simulink model "model"  (R2022a)
settings: Solver=VariableStepAuto  StartTime=0.0  StopTime=Inf  RelTol=1e-3
settings Model: Creator=mateu  LastModifiedBy=mateu

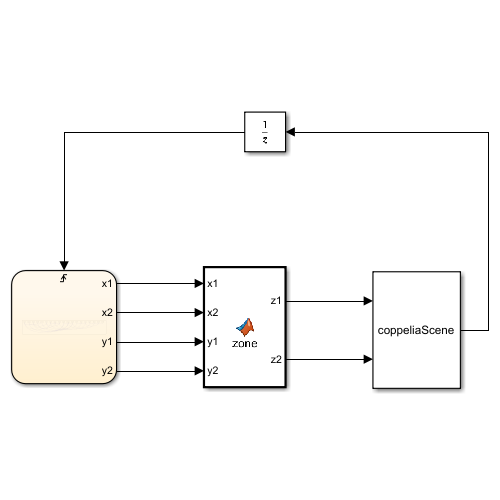
[thumbnail: Simulink's stored preview of the top-level diagram]
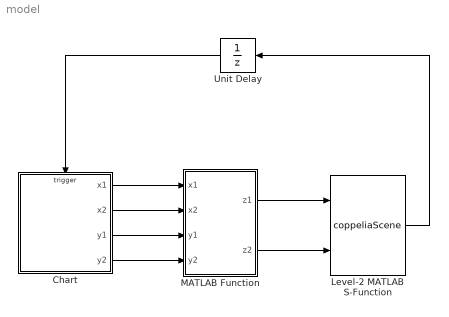
== system model ==
  Chart : Stateflow chart  TreatAsAtomicUnit=on
  Level-2 MATLAB S-Function : M-S-Function  FunctionName=coppeliaScene
  MATLAB Function : MATLAB Function  TreatAsAtomicUnit=on
  Unit Delay : UnitDelay  SampleTime=-1  HasFrameUpgradeWarning=on
  wires:
  MATLAB Function/2(z2) -> Level-2 MATLAB S-Function/2
  MATLAB Function/1(z1) -> Level-2 MATLAB S-Function/1
  Level-2 MATLAB S-Function/1 -> Unit Delay/1
  Chart/1(x1) -> MATLAB Function/1(x1)
  Chart/3(y1) -> MATLAB Function/3(y1)
  Chart/2(x2) -> MATLAB Function/2(x2)
  Chart/4(y2) -> MATLAB Function/4(y2)
  Unit Delay/1 -> Chart/Trigger

== matlab function model/MATLAB Function ==
  data: x1 input; x2 input; z1 output; y1 input; y2 input; z2 output
function [z1,z2] = zone(x1,x2,y1,y2)

z1 = x1 + (y1-1)*3;
z2 = x2 + (y2-1)*3;

== stateflow chart model/Chart ==
  settings: executeAtInitialization=1
  state R_1__x__R_1__y__R_2__x__R_2__y__sup_R_1__S_D__R_1__S_L__R_1__S_R__R_1__S_U__R_1__x__R_1__y__R_2__S_D__R_2__S_L__R_2__S_R__R_2__S_U__R_2__x__R_2__y__S_Collision__S_Task_1___S_Task_2__
    state s01
      x1=1;
      y1=1;
      x2=1;
      y2=2;
    state s02
      x1=1;
      y1=1;
      x2=1;
      y2=2;
    state s03
      x1=1;
      y1=1;
      x2=1;
      y2=3;
    state s04
      x1=1;
      y1=1;
      x2=1;
      y2=3;
    state s05
      x1=1;
      y1=1;
      x2=2;
      y2=1;
    state s06
      x1=1;
      y1=1;
      x2=2;
      y2=1;
    state s07
      x1=1;
      y1=1;
      x2=2;
      y2=1;
    state s08
      x1=1;
      y1=1;
      x2=2;
      y2=2;
    state s09
      x1=1;
      y1=1;
      x2=2;
      y2=2;
    state s010
      x1=1;
      y1=1;
      x2=2;
      y2=3;
    state s011
      x1=1;
      y1=1;
      x2=2;
      y2=3;
    state s012
      x1=1;
      y1=1;
      x2=2;
      y2=3;
    state s013
      x1=1;
      y1=1;
      x2=2;
      y2=3;
    state s014
      x1=1;
      y1=1;
      x2=3;
      y2=1;
    state s015
      x1=1;
      y1=1;
      x2=3;
      y2=1;
    state s016
      x1=1;
      y1=1;
      x2=3;
      y2=1;
    state s017
      x1=1;
      y1=1;
      x2=3;
      y2=2;
    state s018
      x1=1;
      y1=1;
      x2=3;
      y2=2;
    state s019
      x1=1;
      y1=1;
      x2=3;
      y2=3;
    state s020
      x1=1;
      y1=1;
      x2=3;
      y2=3;
    state s021
      x1=1;
      y1=2;
      x2=1;
      y2=1;
    state s022
      x1=1;
      y1=2;
      x2=1;
      y2=1;
    state s023
      x1=1;
      y1=2;
      x2=1;
      y2=3;
    state s024
      x1=1;
      y1=2;
      x2=1;
      y2=3;
    state s025
      x1=1;
      y1=2;
      x2=2;
      y2=1;
    state s026
      x1=1;
      y1=2;
      x2=2;
      y2=1;
    state s027
      x1=1;
      y1=2;
      x2=2;
      y2=1;
    state s028
      x1=1;
      y1=2;
      x2=2;
      y2=1;
    state s029
      x1=1;
      y1=2;
      x2=2;
      y2=2;
    state s030
      x1=1;
      y1=2;
      x2=2;
      y2=2;
    state s031
      x1=1;
      y1=2;
      x2=2;
      y2=3;
    state s032
      x1=1;
      y1=2;
      x2=2;
      y2=3;
    state s033
      x1=1;
      y1=2;
      x2=2;
      y2=3;
    state s034
      x1=1;
      y1=2;
      x2=2;
      y2=3;
    state s035
      x1=1;
      y1=2;
      x2=3;
      y2=1;
    state s036
      x1=1;
      y1=2;
      x2=3;
      y2=1;
    state s037
      x1=1;
      y1=2;
      x2=3;
      y2=2;
    state s038
      x1=1;
      y1=2;
      x2=3;
      y2=2;
    state s039
      x1=1;
      y1=2;
      x2=3;
      y2=3;
    state s040
      x1=1;
      y1=2;
      x2=3;
      y2=3;
    state s041
      x1=1;
      y1=3;
      x2=1;
      y2=1;
    state s042
      x1=1;
      y1=3;
      x2=1;
      y2=2;
    state s043
      x1=1;
      y1=3;
      x2=2;
      y2=1;
    state s044
      x1=1;
      y1=3;
      x2=2;
      y2=1;
    state s045
      x1=1;
      y1=3;
      x2=2;
      y2=2;
    state s046
      x1=1;
      y1=3;
      x2=2;
      y2=3;
    state s047
      x1=1;
      y1=3;
      x2=2;
      y2=3;
    state s048
      x1=1;
      y1=3;
      x2=3;
      y2=1;
    state s049
      x1=1;
      y1=3;
      x2=3;
      y2=2;
    state s050
      x1=1;
      y1=3;
      x2=3;
      y2=3;
    state s051
      x1=2;
      y1=1;
      x2=1;
      y2=1;
    state s052
      x1=2;
      y1=1;
      x2=1;
      y2=2;
    state s053
      x1=2;
      y1=1;
      x2=1;
      y2=3;
    state s054
      x1=2;
      y1=1;
      x2=2;
      y2=2;
    state s055
      x1=2;
      y1=1;
      x2=2;
      y2=3;
    state s056
      x1=2;
      y1=1;
      x2=2;
      y2=3;
    state s057
      x1=2;
      y1=1;
      x2=3;
      y2=1;
    state s058
      x1=2;
      y1=1;
      x2=3;
      y2=1;
    state s059
      x1=2;
      y1=1;
      x2=3;
      y2=2;
    state s060
      x1=2;
      y1=1;
      x2=3;
      y2=3;
    state s061
      x1=2;
      y1=2;
      x2=1;
      y2=1;
    state s062
      x1=2;
      y1=2;
      x2=1;
      y2=2;
    state s063
      x1=2;
      y1=2;
      x2=1;
      y2=3;
    state s064
      x1=2;
      y1=2;
      x2=2;
      y2=1;
    state s065
      x1=2;
      y1=2;
      x2=2;
      y2=1;
    state s066
      x1=2;
      y1=2;
      x2=2;
      y2=3;
    state s067
      x1=2;
      y1=2;
      x2=2;
      y2=3;
    state s068
      x1=2;
      y1=2;
      x2=3;
      y2=1;
    state s069
      x1=2;
      y1=2;
      x2=3;
      y2=2;
    state s070
      x1=2;
      y1=2;
      x2=3;
      y2=3;
    state s071
      x1=2;
      y1=3;
      x2=1;
      y2=1;
    state s072
      x1=2;
      y1=3;
      x2=1;
      y2=2;
    state s073
      x1=2;
      y1=3;
      x2=1;
      y2=3;
    state s074
      x1=2;
      y1=3;
      x2=2;
      y2=1;
    state s075
      x1=2;
      y1=3;
      x2=2;
      y2=1;
    state s076
      x1=2;
      y1=3;
      x2=2;
      y2=2;
    state s077
      x1=2;
      y1=3;
      x2=3;
      y2=1;
    state s078
      x1=2;
      y1=3;
      x2=3;
      y2=2;
    state s079
      x1=2;
      y1=3;
      x2=3;
      y2=3;
    state s080
      x1=3;
      y1=1;
      x2=1;
      y2=1;
    state s081
      x1=3;
      y1=1;
      x2=1;
      y2=2;
    state s082
      x1=3;
      y1=1;
      x2=1;
      y2=3;
    state s083
      x1=3;
      y1=1;
      x2=2;
      y2=1;
    state s084
      x1=3;
      y1=1;
      x2=2;
      y2=1;
    state s085
      x1=3;
      y1=1;
      x2=2;
      y2=2;
    state s086
      x1=3;
      y1=1;
      x2=2;
      y2=3;
    state s087
      x1=3;
      y1=1;
      x2=2;
      y2=3;
    state s088
      x1=3;
      y1=1;
      x2=3;
      y2=2;
    state s089
      x1=3;
      y1=1;
      x2=3;
      y2=3;
    state s090
      x1=3;
      y1=2;
      x2=1;
      y2=1;
    state s091
      x1=3;
      y1=2;
      x2=1;
      y2=1;
    state s092
      x1=3;
      y1=2;
      x2=1;
      y2=2;
    state s093
      x1=3;
      y1=2;
      x2=1;
      y2=2;
    state s094
      x1=3;
      y1=2;
      x2=1;
      y2=3;
    state s095
      x1=3;
      y1=2;
      x2=1;
      y2=3;
    state s096
      x1=3;
      y1=2;
      x2=2;
      y2=1;
    state s097
      x1=3;
      y1=2;
      x2=2;
      y2=1;
    state s098
      x1=3;
      y1=2;
      x2=2;
      y2=1;
    state s099
      x1=3;
      y1=2;
      x2=2;
      y2=1;
    state s0100
      x1=3;
      y1=2;
      x2=2;
      y2=2;
    state s0101
      x1=3;
      y1=2;
      x2=2;
      y2=2;
    state s0102
      x1=3;
      y1=2;
      x2=2;
      y2=3;
    state s0103
      x1=3;
      y1=2;
      x2=2;
      y2=3;
    state s0104
      x1=3;
      y1=2;
      x2=2;
      y2=3;
    state s0105
      x1=3;
      y1=2;
      x2=2;
      y2=3;
    state s0106
      x1=3;
      y1=2;
      x2=3;
      y2=1;
    state s0107
      x1=3;
      y1=2;
      x2=3;
      y2=1;
    state s0108
      x1=3;
      y1=2;
      x2=3;
      y2=3;
    state s0109
      x1=3;
      y1=2;
      x2=3;
      y2=3;
    state s0110
      x1=3;
      y1=3;
      x2=1;
      y2=1;
    state s0111
      x1=3;
      y1=3;
      x2=1;
      y2=2;
    state s0112
      x1=3;
      y1=3;
      x2=1;
      y2=3;
    state s0113
      x1=3;
      y1=3;
      x2=2;
      y2=1;
    state s0114
      x1=3;
      y1=3;
      x2=2;
      y2=1;
    state s0115
      x1=3;
      y1=3;
      x2=2;
      y2=2;
    state s0116
      x1=3;
      y1=3;
      x2=2;
      y2=3;
    state s0117
      x1=3;
      y1=3;
      x2=2;
      y2=3;
    state s0118
      x1=3;
      y1=3;
      x2=3;
      y2=1;
    state s0119
      x1=3;
      y1=3;
      x2=3;
      y2=2;
    (default) -> s014
    s03 -> s01 [order 2] : R2d
    s01 -> s052 : R1r
    s04 -> s02 [order 2] : R2d
    s02 -> s052 : R1r
    s011 -> s03 [order 2] : R2l
    s023 -> s03 : R1d
    s024 -> s03 : R1d
    s03 -> s053 [order 1] : R1r
    s013 -> s04 [order 2] : R2l
    s04 -> s053 [order 1] : R1r
    s025 -> s05 [order 1] : R1d
    s027 -> s05 [order 1] : R1d
    s05 -> s015 : R2r
    s09 -> s06 [order 2] : R2d
    s026 -> s06 [order 1] : R1d
    s028 -> s06 [order 1] : R1d
    s06 -> s015 : R2r
    s08 -> s07 [order 2] : R2d
    s07 -> s016 : R2r
    s012 -> s08 [order 2] : R2d
    s08 -> s054 [order 1] : R1r
    s010 -> s09 [order 2] : R2d
    s029 -> s09 [order 1] : R1d
    s030 -> s09 [order 1] : R1d
    s09 -> s054 [order 1] : R1r
    s019 -> s010 [order 2] : R2l
    s031 -> s010 [order 1] : R1d
    s033 -> s010 [order 1] : R1d
    s010 -> s055 [order 1] : R1r
    s010 -> s011 [order 3] : a2
    s032 -> s011 [order 1] : R1d
    s034 -> s011 [order 1] : R1d
    s011 -> s056 [order 1] : R1r
    s020 -> s012 [order 2] : R2l
    s012 -> s055 [order 1] : R1r
    s012 -> s013 [order 3] : a2
    s013 -> s056 [order 1] : R1r
    s014 -> s057 [order 1] : R1r
    s014 -> s018 [order 2] : R2u
    s035 -> s015 [order 1] : R1d
    s036 -> s015 [order 1] : R1d
    s015 -> s058 [order 1] : R1r
    s015 -> s017 [order 2] : R2u
    s016 -> s058 [order 1] : R1r
    s016 -> s018 [order 2] : R2u
    s037 -> s017 [order 1] : R1d
    s038 -> s017 [order 1] : R1d
    s017 -> s059 [order 1] : R1r
    s017 -> s019 [order 2] : R2u
    s018 -> s059 [order 1] : R1r
    s018 -> s020 [order 2] : R2u
    s039 -> s019 [order 1] : R1d
    s040 -> s019 [order 1] : R1d
    s019 -> s060 [order 1] : R1r
    s020 -> s060 [order 1] : R1r
    s041 -> s021 [order 1] : R1d
    s021 -> s025 : R2r
    s061 -> s022 [order 1] : R1l
    s022 -> s027 : R2r
    s032 -> s023 [order 2] : R2l
    s034 -> s024 [order 2] : R2l
    s063 -> s024 [order 1] : R1l
    s043 -> s025 [order 1] : R1d
    s025 -> s035 [order 2] : R2r
    s029 -> s026 [order 2] : R2d
    s044 -> s026 [order 1] : R1d
    s026 -> s035 [order 2] : R2r
    s064 -> s027 [order 1] : R1l
    s027 -> s036 [order 2] : R2r
    s030 -> s028 [order 2] : R2d
    s065 -> s028 [order 1] : R1l
    s028 -> s036 [order 2] : R2r
    s031 -> s029 [order 2] : R2d
    s045 -> s029 [order 1] : R1d
    s033 -> s030 [order 2] : R2d
    s039 -> s031 [order 2] : R2l
    s046 -> s031 [order 1] : R1d
    s031 -> s032 [order 3] : a2
    s047 -> s032 : R1d
    s040 -> s033 [order 2] : R2l
    s066 -> s033 [order 1] : R1l
    s033 -> s034 [order 3] : a2
    s067 -> s034 [order 1] : R1l
    s048 -> s035 [order 1] : R1d
    s035 -> s037 [order 2] : R2u
    s068 -> s036 [order 1] : R1l
    s036 -> s038 [order 2] : R2u
    s049 -> s037 [order 1] : R1d
    s037 -> s039 [order 2] : R2u
    s069 -> s038 [order 1] : R1l
    s038 -> s040 [order 2] : R2u
    s050 -> s039 [order 1] : R1d
    s070 -> s040 [order 1] : R1l
    s042 -> s041 : R2d
    s071 -> s041 [order 1] : R1l
    s041 -> s043 [order 2] : R2r
    s072 -> s042 [order 1] : R1l
    s074 -> s043 [order 1] : R1l
    s043 -> s048 [order 2] : R2r
    s045 -> s044 [order 2] : R2d
    s075 -> s044 [order 1] : R1l
    s044 -> s048 [order 2] : R2r
    s046 -> s045 [order 2] : R2d
    s076 -> s045 [order 1] : R1l
    s050 -> s046 [order 2] : R2l
    s046 -> s047 [order 3] : a2
    s077 -> s048 [order 1] : R1l
    s048 -> s049 [order 2] : R2u
    s078 -> s049 [order 1] : R1l
    s049 -> s050 [order 2] : R2u
    s079 -> s050 : R1l
    s052 -> s051 [order 2] : R2d
    s051 -> s080 : R1r
    s053 -> s052 [order 2] : R2d
    s052 -> s081 [order 1] : R1r
    s056 -> s053 [order 2] : R2l
    s053 -> s082 [order 1] : R1r
    s055 -> s054 [order 2] : R2d
    s054 -> s085 : R1r
    s060 -> s055 [order 2] : R2l
    s055 -> s086 [order 1] : R1r
    s055 -> s056 [order 3] : a2
    s056 -> s087 [order 1] : R1r
    s057 -> s059 : R2u
    s058 -> s059 : R2u
    s059 -> s088 [order 1] : R1r
    s059 -> s060 [order 2] : R2u
    s060 -> s089 [order 1] : R1r
    s062 -> s061 : R2d
    s090 -> s061 [order 1] : R1l
    s061 -> s064 [order 2] : R2r
    s063 -> s062 [order 2] : R2d
    s092 -> s062 [order 1] : R1l
    s067 -> s063 [order 2] : R2l
    s094 -> s063 [order 1] : R1l
    s096 -> s064 [order 1] : R1l
    s064 -> s068 [order 2] : R2r
    s098 -> s065 [order 1] : R1l
    s065 -> s068 [order 2] : R2r
    s070 -> s066 [order 2] : R2l
    s0102 -> s066 [order 1] : R1l
    s066 -> s067 [order 2] : a2
    s0103 -> s067 [order 1] : R1l
    s0106 -> s068 [order 1] : R1l
    s068 -> s069 [order 2] : R2u
    s069 -> s070 [order 2] : R2u
    s0108 -> s070 [order 1] : R1l
    s072 -> s071 [order 2] : R2d
    s0110 -> s071 [order 1] : R1l
    s071 -> s074 [order 2] : R2r
    s073 -> s072 : R2d
    s0111 -> s072 [order 1] : R1l
    s0112 -> s073 [order 1] : R1l
    s0113 -> s074 [order 1] : R1l
    s074 -> s077 [order 2] : R2r
    s076 -> s075 [order 2] : R2d
    s0114 -> s075 [order 1] : R1l
    s075 -> s077 [order 2] : R2r
    s0115 -> s076 [order 1] : R1l
    s0118 -> s077 [order 1] : R1l
    s077 -> s078 [order 2] : R2u
    s0119 -> s078 : R1l
    s078 -> s079 [order 2] : R2u
    s081 -> s080 [order 2] : R2d
    s080 -> s090 [order 1] : R1u
    s080 -> s083 [order 2] : R2r
    s082 -> s081 [order 2] : R2d
    s081 -> s092 [order 1] : R1u
    s087 -> s082 [order 2] : R2l
    s082 -> s094 [order 1] : R1u
    s083 -> s096 : R1u
    s085 -> s084 [order 2] : R2d
    s084 -> s098 : R1u
    s086 -> s085 [order 2] : R2d
    s085 -> s0100 [order 1] : R1u
    s089 -> s086 [order 2] : R2l
    s086 -> s0102 [order 1] : R1u
    s086 -> s087 [order 3] : a2
    s087 -> s0103 [order 1] : R1u
    s088 -> s089 : R2u
    s089 -> s0108 [order 1] : R1u
    s092 -> s090 [order 2] : R2d
    s090 -> s096 [order 2] : R2r
    s090 -> s091 [order 3] : a1
    s093 -> s091 [order 2] : R2d
    s091 -> s0110 [order 1] : R1u
    s091 -> s097 [order 2] : R2r
    s094 -> s092 [order 2] : R2d
    s092 -> s093 [order 3] : a1
    s095 -> s093 [order 2] : R2d
    s093 -> s0111 [order 1] : R1u
    s0103 -> s094 [order 2] : R2l
    s094 -> s095 [order 3] : a1
    s0105 -> s095 [order 2] : R2l
    s095 -> s0112 [order 1] : R1u
    s096 -> s0106 [order 2] : R2r
    s096 -> s097 [order 3] : a1
    s097 -> s0113 [order 1] : R1u
    s097 -> s0107 [order 2] : R2r
    s0100 -> s098 [order 1] : R2d
    s098 -> s0106 [order 2] : R2r
    s098 -> s099 [order 3] : a1
    s0101 -> s099 [order 2] : R2d
    s099 -> s0114 [order 1] : R1u
    s099 -> s0107 [order 2] : R2r
    s0102 -> s0100 [order 2] : R2d
    s0100 -> s0101 [order 2] : a1
    s0104 -> s0101 [order 2] : R2d
    s0101 -> s0115 [order 1] : R1u
    s0108 -> s0102 [order 2] : R2l
    s0102 -> s0104 [order 3] : a1
    s0102 -> s0103 [order 4] : a2
    s0103 -> s0105 [order 3] : a1
    s0109 -> s0104 : R2l
    s0104 -> s0116 [order 1] : R1u
    s0104 -> s0105 [order 3] : a2
    s0105 -> s0117 [order 1] : R1u
    s0106 -> s0107 [order 2] : a1
    s0107 -> s0118 : R1u
    s0108 -> s0109 [order 3] : a1
    s0111 -> s0110 [order 2] : R2d
    s0110 -> s0113 [order 2] : R2r
    s0112 -> s0111 [order 2] : R2d
    s0117 -> s0112 : R2l
    s0113 -> s0118 [order 2] : R2r
    s0115 -> s0114 [order 2] : R2d
    s0114 -> s0118 [order 2] : R2r
    s0116 -> s0115 [order 1] : R2d
    s0116 -> s0117 [order 2] : a2
    s0118 -> s0119 [order 2] : R2u
  (default) -> R_1__x__R_1__y__R_2__x__R_2__y__sup_R_1__S_D__R_1__S_L__R_1__S_R__R_1__S_U__R_1__x__R_1__y__R_2__S_D__R_2__S_L__R_2__S_R__R_2__S_U__R_2__x__R_2__y__S_Collision__S_Task_1___S_Task_2__
  data: x1 output; x2 output; y1 output; y2 output
  events: R1d input RISING_EDGE_EVENT; R1l input RISING_EDGE_EVENT; R1r input RISING_EDGE_EVENT; R1u input RISING_EDGE_EVENT; R2d input RISING_EDGE_EVENT; R2l input RISING_EDGE_EVENT; R2r input RISING_EDGE_EVENT; R2u input RISING_EDGE_EVENT; a1 input RISING_EDGE_EVENT; a2 input RISING_EDGE_EVENT
